simulink model "Model_1"  (R2020b)
settings: Solver=FixedStepDiscrete  StartTime=0.0  StopTime=10.0  RelTol=1e-3
libraries: dspsrcs4 x1
settings Model: Creator=Diwakar Reddy  LastModifiedBy=Diwakar Reddy

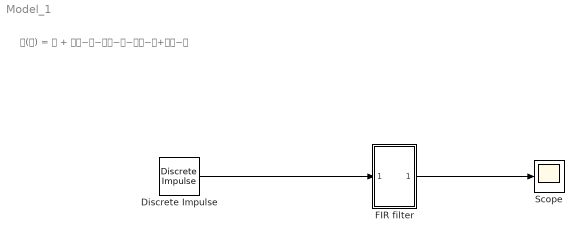
== system Model_1 ==
  note: 𝐇(𝐳) = 𝟏 + 𝟐𝐳−𝟏−𝟑𝐳−𝟐−𝟒𝐳−𝟑+𝟓𝐳−𝟒
  Discrete Impulse : dspsrcs4/Discrete  Impulse  Delay=0  SampleTime=1  FrameSample=1  OutputFrames=off  dataType=double  isSigned=on  wordLen=16  udDataType=sfix(16)  fracBitsMode=Best precision  numFracBits=15  OutDataTypeStr=double  LastOutDataTypeStr=double
  FIR filter : Subsystem
  Scope : Scope
  wires:
  Discrete Impulse/1 -> FIR filter/1(In1)
  FIR filter/1(Out1) -> Scope/1

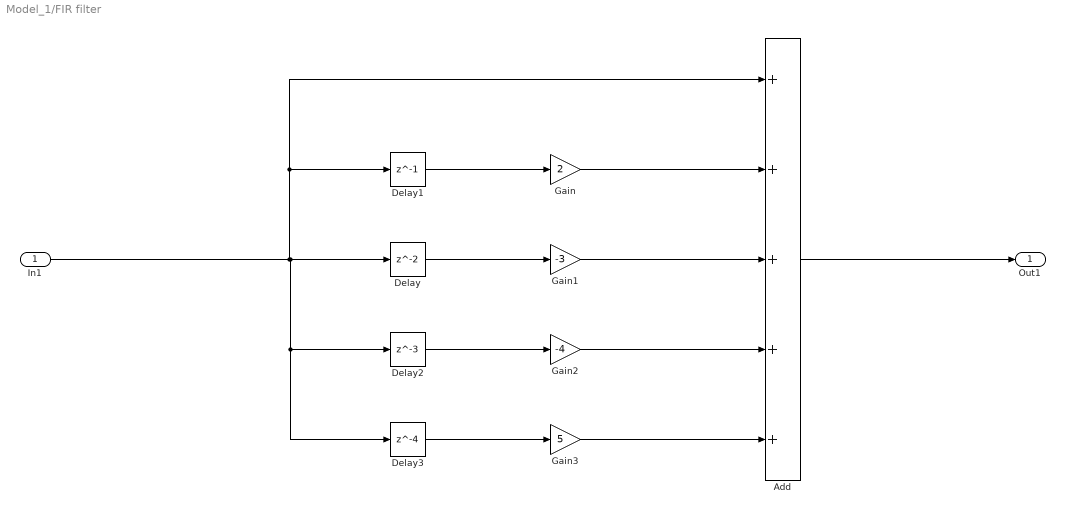
== system Model_1/FIR filter ==
  In1 : Inport
  Add : Sum  Inputs=+++++
  Delay : Delay
  Delay1 : Delay  DelayLength=1
  Delay2 : Delay  DelayLength=3
  Delay3 : Delay  DelayLength=4
  Gain : Gain  Gain=2
  Gain1 : Gain  Gain=-3
  Gain2 : Gain  Gain=-4
  Gain3 : Gain  Gain=5
  Out1 : Outport
  wires:
  Gain3/1 -> Add/5
  Delay2/1 -> Gain2/1
  Gain1/1 -> Add/3
  In1/1 -> Add/1, Delay1/1, Delay3/1, Delay2/1, Delay/1
  Gain/1 -> Add/2
  Delay3/1 -> Gain3/1
  Delay/1 -> Gain1/1
  Delay1/1 -> Gain/1
  Gain2/1 -> Add/4
  Add/1 -> Out1/1
